simulink library "common_lib"  (R2023a)
settings: Solver=ode45  StartTime=0.0  StopTime=10.0  RelTol=1e-3
undefined symbols (not defined in the file): ACCEL_PRE_MULT, APDT_SrvcMgr_IRVHVDCSubFcnReq, C_C1GearNumbers, C_C1GearRatios, C_Calibration, C_DitherWaveform, C_GearOffset, C_GearRatioIn, C_GearRatioInverseOut, C_GearRatioOut, CLUTCH_INNER_LOOP_UPDATE_RATE, CONSTANT, DEGRADED_MODE_SIZE, Dem_EventStatusType, DiscIntNeverNeededParam, F_FAULT_ENUM, F_NOFAULT, F_OUTOFRANGE, F_RATELIMIT, FALSE, FMI14_SPECIAL_INSTRUCTIONS, FMI20_DATA_DRIFTED_HIGH, FMI21_DATA_DRIFTED_LOW, FMI29_RESERVED_FOR_SAE_ASSIGNMENT, FMI30_RESERVED_FOR_SAE_ASSIGNMENT, FMI31_CONDITION_EXISTS, FMI32_NO_FAULT, IC, k_accel, k_mean, MAX_UINT32, MEAN_PRE_MULT, NTriggers, QLTY_SIGNAL_FAILED, QLTY_SIGNAL_FULLY_FUNCTION, QLTY_SIGNAL_SUBSTITUTED_BY_1ST_CHOICE, QLTY_SIGNAL_SUBSTITUTED_BY_2ND_CHOICE, QLTY_SIGNAL_SUBSTITUTED_BY_3RD_CHOICE, QLTY_SIGNAL_SUBSTITUTED_BY_4TH_CHOICE, SAMPLE_TIME_100us, SAMPLETIME_10ms_Int, SATURATION_U16, simin, T_TestPoint, TF_FALSE, TF_TRUE, TimeStep, TRUE, WORKSPACE_UPDATE_RATE, ZERO, Zero
libraries: $bdroot x123, simulink x28, simulink_extras x4, MBD_EPS_Local_Blockset x4
(part 9 of 10)

== system common_lib/Diag/Fault Counter/FaultCounter ==
  fl : Inport
  count_prev : Inport  Port=2
  fc_level : Inport  Port=3
  reset : Inport  Port=4  OutDataTypeStr=boolean
  Enable : EnablePort  ZeroCross=off
  Constant1 : Constant  Value=ZERO
  Constant2 : Constant  Value=false
  Constant3 : Constant  Value=true
  Constant6 : Constant  Value=ZERO
  Relay : $bdroot/Slink/Relay  init=false
      settings: AttributesFormatString=ic=%<init>
  Sat : $bdroot/Slink/Sat
  Sum : Sum  Inputs=++|  InputSameDT=on  OutDataTypeStr=Inherit: Same as first input
  reset switch1 : Switch  Criteria=u2 ~= 0  Threshold=0.5  ZeroCross=off  SaturateOnIntegerOverflow=off
  count : Outport  OutputWhenDisabled=reset  InitialOutput=ZERO  VectorParamsAs1DForOutWhenUnconnected=off
  fc : Outport  Port=2  OutputWhenDisabled=reset  InitialOutput=false  VectorParamsAs1DForOutWhenUnconnected=off
  wires:
  Sum/1 -> reset switch1/3
  Constant6/1 -> reset switch1/1
  Relay/1 -> fc/1
  Constant3/1 -> Relay/4
  Constant2/1 -> Relay/5
  Constant1/1 -> Relay/3, Sat/3
  fc_level/1 -> Relay/2, Sat/2
  fl/1 -> Sum/2
  reset/1 -> reset switch1/2
  reset switch1/1 -> Relay/1, Sat/1
  count_prev/1 -> Sum/1
  Sat/1 -> count/1

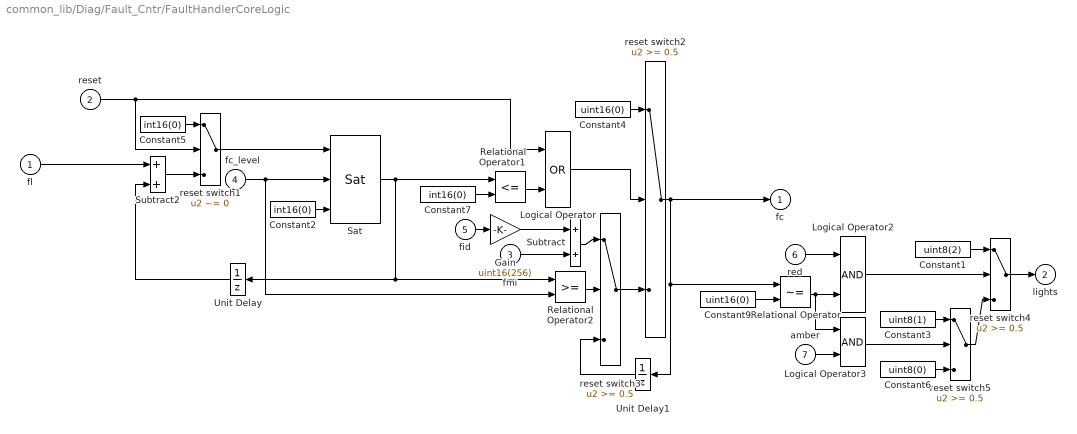
== system common_lib/Diag/Fault_Cntr/FaultHandlerCoreLogic ==
  fl : Inport  OutDataTypeStr=int16
  reset : Inport  Port=2  OutDataTypeStr=boolean
  fmi : Inport  Port=3  OutDataTypeStr=uint16
  fc_level : Inport  Port=4  OutDataTypeStr=int16
  fid : Inport  Port=5  OutDataTypeStr=uint16
  red : Inport  Port=6  OutDataTypeStr=boolean
  amber : Inport  Port=7  OutDataTypeStr=boolean
  Constant1 : Constant  Value=uint8(2)
  Constant2 : Constant  Value=int16(0)
  Constant3 : Constant  Value=uint8(1)
  Constant4 : Constant  Value=uint16(0)
  Constant5 : Constant  Value=int16(0)
  Constant6 : Constant  Value=uint8(0)
  Constant7 : Constant  Value=int16(0)
  Constant9 : Constant  Value=uint16(0)
  Gain : Gain  Gain=uint16(256)
  Logical Operator : Logic  Operator=OR  AllPortsSameDT=off  OutDataTypeStr=boolean
  Logical Operator2 : Logic  AllPortsSameDT=off  OutDataTypeStr=boolean
  Logical Operator3 : Logic  AllPortsSameDT=off  OutDataTypeStr=boolean
  Relational Operator : RelationalOperator  Operator=~=  OutDataTypeStr=boolean  InputSameDT=off
  Relational Operator1 : RelationalOperator  Operator=<=  OutDataTypeStr=boolean  InputSameDT=off
  Relational Operator2 : RelationalOperator  OutDataTypeStr=boolean  InputSameDT=off
  Sat : $bdroot/Slink/Sat
  Subtract : Sum  OutDataTypeStr=uint16
  Subtract2 : Sum  OutDataTypeStr=int16  SaturateOnIntegerOverflow=on
  Unit Delay : UnitDelay  InitialCondition=int16(0)  SampleTime=-1  HasFrameUpgradeWarning=on
      settings: AttributesFormatString=ic=%<X0>
  Unit Delay1 : UnitDelay  InitialCondition=uint16(0)  SampleTime=-1  HasFrameUpgradeWarning=on
      settings: AttributesFormatString=ic=%<X0>
  reset switch1 : Switch  Criteria=u2 ~= 0  Threshold=0.5  ZeroCross=off  SaturateOnIntegerOverflow=off
  reset switch{2..5} (4 alike) : Switch  Threshold=0.5  ZeroCross=off  SaturateOnIntegerOverflow=off
  fc : Outport  VectorParamsAs1DForOutWhenUnconnected=off
  lights : Outport  Port=2  VectorParamsAs1DForOutWhenUnconnected=off
  wires:
  Gain/1 -> Subtract/1
  reset switch3/1 -> reset switch2/3
  Unit Delay1/1 -> reset switch3/3
  Relational Operator2/1 -> reset switch3/2
  Relational Operator1/1 -> Logical Operator/2
  Constant7/1 -> Relational Operator1/2
  Unit Delay/1 -> Subtract2/2
  Subtract2/1 -> reset switch1/3
  reset switch1/1 -> Sat/1
  Constant5/1 -> reset switch1/1
  reset switch2/1 -> Unit Delay1/1, Relational Operator/1, fc/1
  Logical Operator/1 -> reset switch2/2
  Subtract/1 -> reset switch3/1
  Constant4/1 -> reset switch2/1
  fmi/1 -> Subtract/2
  fid/1 -> Gain/1
  reset/1 -> Logical Operator/1, reset switch1/2
  fl/1 -> Subtract2/1
  Sat/1 -> Relational Operator2/1, Unit Delay/1, Relational Operator1/1
  Constant9/1 -> Relational Operator/2
  Logical Operator2/1 -> reset switch4/2
  Relational Operator/1 -> Logical Operator2/2, Logical Operator3/1
  red/1 -> Logical Operator2/1
  amber/1 -> Logical Operator3/2
  fc_level/1 -> Sat/2, Relational Operator2/2
  Constant2/1 -> Sat/3
  Constant1/1 -> reset switch4/1
  Logical Operator3/1 -> reset switch5/2
  reset switch5/1 -> reset switch4/3
  Constant3/1 -> reset switch5/1
  Constant6/1 -> reset switch5/3
  reset switch4/1 -> lights/1

== system common_lib/Diag/Filter w Fault Handler/FilterWithFaultHandlerCoreLogic ==
  note: Common Library::Diagnostics::Filter With Fault Handler
  input : Inport
  tau : Inport  Port=2
  override_value : Inport  Port=3
  override? : Inport  Port=4
  reset? : Inport  Port=5
  default : Inport  Port=6
  ramp_time : Inport  Port=7
  fault? : Inport  Port=8
  Abs1 : Abs  ZeroCross=off  SaturateOnIntegerOverflow=off
  Abs2 : Abs  ZeroCross=off  SaturateOnIntegerOverflow=off
  Constant5 : Constant  Value=TimeStep
  Data Type Conversion : DataTypeConversion  OutDataTypeStr=single  SaturateOnIntegerOverflow=off  RndMeth=Floor
  Fltr_wRO : $bdroot/Fltrs/Fltr_wRO  TimeStep=TimeStep
  Product1 : Product  Inputs=**/  InputSameDT=on  OutDataTypeStr=Inherit: Same as first input
  Sum1 : Sum  Inputs=+-|  InputSameDT=on  OutDataTypeStr=Inherit: Same as first input
  Sum2 : Sum  Inputs=+-|  InputSameDT=on  OutDataTypeStr=Inherit: Same as first input
  Sum3 : Sum  Inputs=+-|  InputSameDT=on  OutDataTypeStr=Inherit: Same as first input
  Switch{1..4} (4 alike) : Switch  Threshold=0.5  ZeroCross=off  SaturateOnIntegerOverflow=off
  delay : UnitDelay  InitialCondition=Zero  SampleTime=-1  HasFrameUpgradeWarning=on
  ic: signal at fault : UnitDelay  InitialCondition=Zero  SampleTime=-1  HasFrameUpgradeWarning=on
  within zero tol of corrections : RelationalOperator  Operator=<  ZeroCross=off  InputSameDT=off
  output : Outport  VectorParamsAs1DForOutWhenUnconnected=off
  wires:
  Data Type Conversion/1 -> Product1/2
  Constant5/1 -> Data Type Conversion/1
  Sum3/1 -> Abs1/1
  delay/1 -> Switch2/1
  Switch3/1 -> delay/1
  within zero tol of corrections/1 -> Switch3/2
  Abs2/1 -> within zero tol of corrections/1
  Abs1/1 -> within zero tol of corrections/2
  Sum2/1 -> Switch3/1
  Switch1/1 -> Sum3/1, Sum2/1
  Switch4/1 -> Switch1/3, Sum1/1, ic: signal at fault/1
  ic: signal at fault/1 -> Switch4/1
  Product1/1 -> Abs2/1, Sum2/2
  Sum1/1 -> Product1/1
  default/1 -> Sum3/2, Switch3/3, Sum1/2
  Fltr_wRO/1 -> Switch4/3, output/1
  input/1 -> Switch2/3
  Switch2/1 -> Switch1/1, Fltr_wRO/1
  reset?/1 -> Fltr_wRO/5
  override?/1 -> Fltr_wRO/4
  override_value/1 -> Fltr_wRO/3
  tau/1 -> Fltr_wRO/2
  fault?/1 -> Switch1/2, Switch4/2, Switch2/2
  ramp_time/1 -> Product1/3

== system common_lib/Diag/Filter w Fault Handler1/Fltr_wRO ==
  note: This is a simple 1st order filter block with reset and override.
      |
      |      If override is true (1) then output=override_value
      |      If       reset is true (1) then output=input
      |    otherwise output = previous output + (input - previous output) * T/tau
  note: Common Library::Filters::Filter with Reset and Override
  input : Inport
  tau : Inport  Port=2
  reset? : Inport  Port=3  OutDataTypeStr=boolean
  Constant1 : Constant  Value=TimeStep
  Constant3 : Constant  Value=TimeStep
  MinMax : MinMax  Function=max  Inputs=2  InputSameDT=on  SaturateOnIntegerOverflow=on  ZeroCross=off
  Product : Product  Inputs=**/  InputSameDT=on  OutDataTypeStr=Inherit: Same as first input
  Sum : Sum  Inputs=|+-  InputSameDT=on  OutDataTypeStr=Inherit: Same as first input
  Sum1 : Sum  Inputs=|++  InputSameDT=on  OutDataTypeStr=Inherit: Same as first input
  Switch2 : Switch  Threshold=0.5  ZeroCross=off  SaturateOnIntegerOverflow=off
  Unit Delay : UnitDelay  InitialCondition=IC  SampleTime=-1  HasFrameUpgradeWarning=on
  output : Outport  VectorParamsAs1DForOutWhenUnconnected=off
  wires:
  Sum1/1 -> Switch2/3
  Product/1 -> Sum1/1
  tau/1 -> MinMax/2
  Constant1/1 -> MinMax/1
  Unit Delay/1 -> Sum1/2, Sum/2
  input/1 -> Switch2/1, Sum/1
  Constant3/1 -> Product/2
  MinMax/1 -> Product/3
  reset?/1 -> Switch2/2
  Sum/1 -> Product/1
  Switch2/1 -> Unit Delay/1, output/1

== system common_lib/Diagnostics/CAN OOR Fault Detection/detect fault ==
  In1 : Inport
  Enable : EnablePort
  Data Type Conversion Inherited : simulink/Signal Attributes/Data Type Conversion Inherited  ConvertRealWorld=Real World Value  RndMeth=Ceiling  DoSatur=off
  Data Type Conversion Inherited1 : simulink/Signal Attributes/Data Type Conversion Inherited  ConvertRealWorld=Real World Value  RndMeth=Ceiling  DoSatur=off
  Logical Operator : Logic  Operator=OR  AllPortsSameDT=off  OutDataTypeStr=boolean
  Relational Operator : RelationalOperator  Operator=<  OutDataTypeStr=boolean  ZeroCross=off  InputSameDT=off
  Relational Operator1 : RelationalOperator  Operator=<  OutDataTypeStr=boolean  ZeroCross=off  InputSameDT=off
  max : Constant  Value=k_max
  min : Constant  Value=k_min
  fault set : Outport
  wires:
  Relational Operator1/1 -> Logical Operator/1
  Relational Operator/1 -> Logical Operator/2
  Logical Operator/1 -> fault set/1
  Data Type Conversion Inherited/1 -> Relational Operator1/1
  Data Type Conversion Inherited1/1 -> Relational Operator/2
  min/1 -> Data Type Conversion Inherited1/2
  max/1 -> Data Type Conversion Inherited/2
  In1/1 -> Data Type Conversion Inherited1/1, Relational Operator1/2, Relational Operator/1, Data Type Conversion Inherited/1

== system common_lib/Diagnostics/Calibration Enabled MinMax OOR/Enabled OOR ==
  In : Inport
  ULim : Inport  Port=2
  LLim : Inport  Port=3
  Ext_Fault : Inport  Port=4
  Enable : EnablePort  ZeroCross=off
      settings: AttributesFormatString=%<StatesWhenEnabling>
  Calibration with Pretty Print Value : $bdroot/IO/Calibration with Pretty Print Value  CalValue=C_IMgmt_OOR_MinMaxCapture_Enable  scaling=None
  OOR Fault Detection : $bdroot/Diag/OOR Fault Detection  InitialValue=InitialValue
  OOR MinMax Capture : Subsystem
  Out : Outport  InitialOutput=0  VectorParamsAs1DForOutWhenUnconnected=off
      settings: AttributesFormatString=|
      | OutputWhenDisabled=%<OutputWhenDisabled>
      | InitialOutput=%<InitialOutput>
  Fault : Outport  Port=2  InitialOutput=0  VectorParamsAs1DForOutWhenUnconnected=off
      settings: AttributesFormatString=|
      | OutputWhenDisabled=%<OutputWhenDisabled>
      | InitialOutput=%<InitialOutput>
  Max : Outport  Port=3  VectorParamsAs1DForOutWhenUnconnected=off
      settings: AttributesFormatString=|
      | OutputWhenDisabled=%<OutputWhenDisabled>
      | InitialOutput=%<InitialOutput>
  Min : Outport  Port=4  VectorParamsAs1DForOutWhenUnconnected=off
      settings: AttributesFormatString=|
      | OutputWhenDisabled=%<OutputWhenDisabled>
      | InitialOutput=%<InitialOutput>
  wires:
  LLim/1 -> OOR Fault Detection/3
  ULim/1 -> OOR Fault Detection/2
  In/1 -> OOR Fault Detection/1, OOR MinMax Capture/1(Input)
  Ext_Fault/1 -> OOR Fault Detection/4, OOR MinMax Capture/2(Hold)
  OOR Fault Detection/1 -> Out/1
  OOR Fault Detection/2 -> Fault/1
  OOR MinMax Capture/1(Max) -> Max/1
  OOR MinMax Capture/2(Min) -> Min/1
  Calibration with Pretty Print Value/1 -> OOR MinMax Capture/Enable

== system common_lib/Diagnostics/Calibration Enabled MinMax RLim/Enabled RLim ==
  In : Inport
  RLim : Inport  Port=2
  Ext_Fault : Inport  Port=3
  Enable : EnablePort  ZeroCross=off
      settings: AttributesFormatString=%<StatesWhenEnabling>
  Calibration with Pretty Print Value : $bdroot/IO/Calibration with Pretty Print Value  CalValue=C_IMgmt_RLim_MinMaxCapture_Enable  scaling=None
  Data Type Conversion : DataTypeConversion  OutDataTypeStr=single  SaturateOnIntegerOverflow=off  RndMeth=Floor
  Data Type Conversion1 : DataTypeConversion  OutDataTypeStr=single  SaturateOnIntegerOverflow=off  RndMeth=Floor
  RLim MinMax Capture : Subsystem
  RateLimit : Subsystem  mask{IC=IC, TimeStep=TimeStep}
      mask prompts: IC "Initial Condition"; TimeStep "Update Time"
  out : Outport  VectorParamsAs1DForOutWhenUnconnected=off
      settings: AttributesFormatString=|
      | OutputWhenDisabled=%<OutputWhenDisabled>
      | InitialOutput=%<InitialOutput>
  fault? : Outport  Port=2  VectorParamsAs1DForOutWhenUnconnected=off
      settings: AttributesFormatString=|
      | OutputWhenDisabled=%<OutputWhenDisabled>
      | InitialOutput=%<InitialOutput>
  Max Pos Rate : Outport  Port=3  VectorParamsAs1DForOutWhenUnconnected=off
      settings: AttributesFormatString=|
      | OutputWhenDisabled=%<OutputWhenDisabled>
      | InitialOutput=%<InitialOutput>
  Max Neg Rate : Outport  Port=4  VectorParamsAs1DForOutWhenUnconnected=off
      settings: AttributesFormatString=|
      | OutputWhenDisabled=%<OutputWhenDisabled>
      | InitialOutput=%<InitialOutput>
  wires:
  In/1 -> Data Type Conversion/1, RLim MinMax Capture/1(Input)
  Ext_Fault/1 -> RLim MinMax Capture/2(Hold), RateLimit/3(ext_fault?)
  RateLimit/1(out) -> out/1
  RLim/1 -> Data Type Conversion1/1
  RateLimit/2(fault?) -> fault?/1
  RLim MinMax Capture/2(Min) -> Max Neg Rate/1
  RLim MinMax Capture/1(Max) -> Max Pos Rate/1
  Data Type Conversion/1 -> RateLimit/1(in)
  Data Type Conversion1/1 -> RateLimit/2(rlim)
  Calibration with Pretty Print Value/1 -> RLim MinMax Capture/Enable

== system common_lib/Diagnostics/DiagDbncCntr/Counter1 ==
  note: Counter increments when "incr condition" is TRUE and decrements when "decr condition" is TRUE.
  note: Common Library::Miscellaneous::Counter
  up_val : Inport
  count_up? : Inport  Port=2  OutDataTypeStr=boolean
  down_val : Inport  Port=3
  count_down? : Inport  Port=4  OutDataTypeStr=boolean
  max_count : Inport  Port=5
  min_count : Inport  Port=6
  reset? : Inport  Port=7  OutDataTypeStr=boolean
  Constant1 : Constant  Value=Zero  OutDataTypeStr=uint16
  Constant2 : Constant  Value=Zero  OutDataTypeStr=uint16
  Constant4 : Constant  Value=IC
  Constant5 : Constant  Value=false
  Logical Operator : Logic  Operator=OR
  Sat : $bdroot/Slink/Sat
  Sum : Sum  Inputs=++-  InputSameDT=on  SaturateOnIntegerOverflow=on  OutDataTypeStr=Inherit: Same as first input
  Unit Delay : UnitDelay  InitialCondition=IC  SampleTime=-1  HasFrameUpgradeWarning=on
  Unit Delay1 : UnitDelay  InitialCondition=true  SampleTime=-1  HasFrameUpgradeWarning=on
  dec switch : Switch  Threshold=0.5  ZeroCross=off  SaturateOnIntegerOverflow=off
  inc switch : Switch  Threshold=0.5  ZeroCross=off  SaturateOnIntegerOverflow=off
  reset switch : Switch  Threshold=0.5  ZeroCross=off  SaturateOnIntegerOverflow=off
  output : Outport  VectorParamsAs1DForOutWhenUnconnected=off
  wires:
  count_down?/1 -> dec switch/2
  down_val/1 -> dec switch/1
  count_up?/1 -> inc switch/2
  up_val/1 -> inc switch/1
  Constant2/1 -> dec switch/3
  dec switch/1 -> Sum/3
  Constant1/1 -> inc switch/3
  inc switch/1 -> Sum/2
  reset?/1 -> Logical Operator/1
  reset switch/1 -> Unit Delay/1, output/1
  Unit Delay/1 -> Sum/1
  Logical Operator/1 -> reset switch/2
  Unit Delay1/1 -> Logical Operator/2
  Constant5/1 -> Unit Delay1/1
  Sat/1 -> reset switch/3
  Constant4/1 -> reset switch/1
  max_count/1 -> Sat/2
  min_count/1 -> Sat/3
  Sum/1 -> Sat/1

== system common_lib/Diagnostics/OOR Fault Detect Enum/detect fault ==
  In1 : Inport
  Enable : EnablePort
  Logical Operator : Logic  Operator=OR  AllPortsSameDT=off  OutDataTypeStr=boolean
  Relational Operator : RelationalOperator  Operator=<  OutDataTypeStr=boolean  ZeroCross=off  InputSameDT=off
  Relational Operator1 : RelationalOperator  Operator=<  OutDataTypeStr=boolean  ZeroCross=off  InputSameDT=off
  max : Constant  Value=k_max
  min : Constant  Value=k_min
  fault set : Outport
  wires:
  Relational Operator1/1 -> Logical Operator/1
  Relational Operator/1 -> Logical Operator/2
  In1/1 -> Relational Operator1/2, Relational Operator/1
  Logical Operator/1 -> fault set/1
  max/1 -> Relational Operator1/1
  min/1 -> Relational Operator/2

== system common_lib/Diagnostics/OOR Fault Detection/detect fault ==
  In1 : Inport
  Enable : EnablePort
  Data Type Conversion Inherited : simulink/Signal Attributes/Data Type Conversion Inherited  ConvertRealWorld=Real World Value  DoSatur=off
  Data Type Conversion Inherited1 : simulink/Signal Attributes/Data Type Conversion Inherited  ConvertRealWorld=Real World Value  DoSatur=off
  Logical Operator : Logic  Operator=OR  AllPortsSameDT=off
  Relational Operator : RelationalOperator  Operator=<  ZeroCross=off  InputSameDT=off
  Relational Operator1 : RelationalOperator  Operator=<  ZeroCross=off  InputSameDT=off
  max : Constant  Value=k_max
  min : Constant  Value=k_min
  fault set : Outport
  wires:
  Logical Operator/1 -> fault set/1
  In1/1 -> Data Type Conversion Inherited1/1, Relational Operator/1, Relational Operator1/2, Data Type Conversion Inherited/1
  Relational Operator/1 -> Logical Operator/2
  Relational Operator1/1 -> Logical Operator/1
  max/1 -> Data Type Conversion Inherited/2
  Data Type Conversion Inherited/1 -> Relational Operator1/1
  min/1 -> Data Type Conversion Inherited1/2
  Data Type Conversion Inherited1/1 -> Relational Operator/2

== system common_lib/Diagnostics/SetFMI/IF_ELSE_LADDER ==
  FMI_in : Inport  OutDataTypeStr=uint8  PortDimensions=1
  Active1 : Inport  Port=2  OutDataTypeStr=boolean  PortDimensions=1
  Active2 : Inport  Port=3  OutDataTypeStr=boolean  PortDimensions=1
  Active3 : Inport  Port=4  OutDataTypeStr=boolean  PortDimensions=1
  Active4 : Inport  Port=5  OutDataTypeStr=boolean  PortDimensions=1
  Active5 : Inport  Port=6  OutDataTypeStr=boolean  PortDimensions=1
  Active6 : Inport  Port=7  OutDataTypeStr=boolean  PortDimensions=1
  Active7 : Inport  Port=8  OutDataTypeStr=boolean  PortDimensions=1
  FMI_1 : Inport  Port=9  OutDataTypeStr=uint8  PortDimensions=1
  FMI_2 : Inport  Port=10  OutDataTypeStr=uint8  PortDimensions=1
  FMI_3 : Inport  Port=11  OutDataTypeStr=uint8  PortDimensions=1
  FMI_4 : Inport  Port=12  OutDataTypeStr=uint8  PortDimensions=1
  FMI_5 : Inport  Port=13  OutDataTypeStr=uint8  PortDimensions=1
  FMI_6 : Inport  Port=14  OutDataTypeStr=uint8  PortDimensions=1
  FMI_7 : Inport  Port=15  OutDataTypeStr=uint8  PortDimensions=1
  Constant1 : Constant  Value=FMI32_NO_FAULT
  Constant7 : Constant  Value=FMI32_NO_FAULT
  Relational Operator : RelationalOperator  Operator=~=  OutDataTypeStr=boolean  InputSameDT=off
  Switch{,1..7} (8 alike) : Switch  Threshold=0.5  SaturateOnIntegerOverflow=off  InputSameDT=off
  FMI_out : Outport  OutDataTypeStr=uint8  PortDimensions=1  VectorParamsAs1DForOutWhenUnconnected=off
  wires:
  Constant1/1 -> Switch7/3
  FMI_in/1 -> Relational Operator/1, Switch/1
  Active6/1 -> Switch6/2
  Switch1/1 -> Switch/3
  FMI_2/1 -> Switch2/1
  Switch4/1 -> Switch3/3
  FMI_5/1 -> Switch5/1
  Switch3/1 -> Switch2/3
  Switch6/1 -> Switch5/3
  Switch/1 -> FMI_out/1
  FMI_4/1 -> Switch4/1
  FMI_7/1 -> Switch7/1
  FMI_3/1 -> Switch3/1
  Switch7/1 -> Switch6/3
  Active4/1 -> Switch4/2
  Switch5/1 -> Switch4/3
  Constant7/1 -> Relational Operator/2
  Switch2/1 -> Switch1/3
  Active2/1 -> Switch2/2
  Active7/1 -> Switch7/2
  Active1/1 -> Switch1/2
  Active3/1 -> Switch3/2
  Active5/1 -> Switch5/2
  FMI_6/1 -> Switch6/1
  FMI_1/1 -> Switch1/1
  Relational Operator/1 -> Switch/2

== system common_lib/Diagnostics/SignalSubstitution/If Action Subsystem ==
  NoSubstitute : Inport
  Action Port : ActionPort
  Constant4 : Constant  Value=QLTY_SIGNAL_FULLY_FUNCTION  SampleTime=-1
  Signal Conversion : SignalConversion  OverrideOpt=off
  Signal : Outport  VectorParamsAs1DForOutWhenUnconnected=off
  Qlty : Outport  Port=2  VectorParamsAs1DForOutWhenUnconnected=off
  wires:
  NoSubstitute/1 -> Signal Conversion/1
  Constant4/1 -> Qlty/1
  Signal Conversion/1 -> Signal/1

== system common_lib/Diagnostics/SignalSubstitution/If Action Subsystem1 ==
  FirstChoice : Inport
  Action Port : ActionPort
  Constant4 : Constant  Value=QLTY_SIGNAL_SUBSTITUTED_BY_1ST_CHOICE  SampleTime=-1
  Signal Conversion : SignalConversion  OverrideOpt=off
  Signal : Outport  VectorParamsAs1DForOutWhenUnconnected=off
  Qlty : Outport  Port=2  VectorParamsAs1DForOutWhenUnconnected=off
  wires:
  Constant4/1 -> Qlty/1
  FirstChoice/1 -> Signal Conversion/1
  Signal Conversion/1 -> Signal/1

== system common_lib/Diagnostics/SignalSubstitution/If Action Subsystem2 ==
  SecondChoice : Inport
  Action Port : ActionPort
  Constant4 : Constant  Value=QLTY_SIGNAL_SUBSTITUTED_BY_2ND_CHOICE  SampleTime=-1
  Signal Conversion : SignalConversion  OverrideOpt=off
  Signal : Outport  VectorParamsAs1DForOutWhenUnconnected=off
  Qlty : Outport  Port=2  VectorParamsAs1DForOutWhenUnconnected=off
  wires:
  Signal Conversion/1 -> Signal/1
  SecondChoice/1 -> Signal Conversion/1
  Constant4/1 -> Qlty/1

== system common_lib/Diagnostics/SignalSubstitution/If Action Subsystem3 ==
  ThirdChoice : Inport
  Action Port : ActionPort
  Constant4 : Constant  Value=QLTY_SIGNAL_SUBSTITUTED_BY_3RD_CHOICE  SampleTime=-1
  Signal Conversion : SignalConversion  OverrideOpt=off
  Signal : Outport  VectorParamsAs1DForOutWhenUnconnected=off
  Qlty : Outport  Port=2  VectorParamsAs1DForOutWhenUnconnected=off
  wires:
  Constant4/1 -> Qlty/1
  ThirdChoice/1 -> Signal Conversion/1
  Signal Conversion/1 -> Signal/1

== system common_lib/Diagnostics/SignalSubstitution/If Action Subsystem4 ==
  FourthChoice : Inport
  Action Port : ActionPort
  Constant4 : Constant  Value=QLTY_SIGNAL_SUBSTITUTED_BY_4TH_CHOICE  SampleTime=-1
  Signal Conversion : SignalConversion  OverrideOpt=off
  Signal : Outport  VectorParamsAs1DForOutWhenUnconnected=off
  Qlty : Outport  Port=2  VectorParamsAs1DForOutWhenUnconnected=off
  wires:
  Signal Conversion/1 -> Signal/1
  FourthChoice/1 -> Signal Conversion/1
  Constant4/1 -> Qlty/1

== system common_lib/Diagnostics/SignalSubstitution/If Action Subsystem5 ==
  FailedValue : Inport
  Action Port : ActionPort
  Constant4 : Constant  Value=QLTY_SIGNAL_FAILED  SampleTime=-1
  Signal Conversion : SignalConversion  OverrideOpt=off
  Signal : Outport  VectorParamsAs1DForOutWhenUnconnected=off
  Qlty : Outport  Port=2  VectorParamsAs1DForOutWhenUnconnected=off
  wires:
  Constant4/1 -> Qlty/1
  FailedValue/1 -> Signal Conversion/1
  Signal Conversion/1 -> Signal/1

== system common_lib/Fltrs/Fltr_wRO/FilterCoreLogic ==
  note: This is a simple 1st order filter block
  input : Inport  OutDataTypeStr=single
  tau : Inport  Port=2  OutDataTypeStr=single
  override_value : Inport  Port=3
  override? : Inport  Port=4  OutDataTypeStr=boolean
  reset? : Inport  Port=5  OutDataTypeStr=boolean
  Constant1 : Constant  Value=Ts
  MinMax : MinMax  Function=max  Inputs=2  InputSameDT=on  SaturateOnIntegerOverflow=on  ZeroCross=off
  Product : Product  Inputs=**/  InputSameDT=on  OutDataTypeStr=Inherit: Same as first input
  Sum : Sum  Inputs=|+-  InputSameDT=on  OutDataTypeStr=Inherit: Same as first input
  Sum1 : Sum  Inputs=|++  InputSameDT=on  OutDataTypeStr=Inherit: Same as first input
  Switch : Switch  Threshold=0.5  ZeroCross=off  SaturateOnIntegerOverflow=off
  Switch2 : Switch  Threshold=0.5  ZeroCross=off  SaturateOnIntegerOverflow=off
  Unit Delay : UnitDelay  InitialCondition=IC  SampleTime=-1  HasFrameUpgradeWarning=on
  output : Outport  OutDataTypeStr=single  VectorParamsAs1DForOutWhenUnconnected=off
  wires:
  Sum1/1 -> Switch2/3
  Product/1 -> Sum1/1
  tau/1 -> MinMax/2
  input/1 -> Sum/1, Switch2/1
  MinMax/1 -> Product/3
  Sum/1 -> Product/1
  Constant1/1 -> MinMax/1, Product/2
  override_value/1 -> Switch/1
  override?/1 -> Switch/2
  Switch/1 -> output/1, Unit Delay/1
  reset?/1 -> Switch2/2
  Switch2/1 -> Switch/3
  Unit Delay/1 -> Sum1/2, Sum/2

== system common_lib/Fltrs/Fltr_wROExtInitCond/FilterCoreLogic ==
  note: This is a simple 1st order filter block
  input : Inport  OutDataTypeStr=single
  tau : Inport  Port=2  OutDataTypeStr=single
  init_cond : Inport  Port=3  OutDataTypeStr=single
  task_rate : Inport  Port=4  OutDataTypeStr=single
  reset : Inport  Port=5  OutDataTypeStr=boolean
  override : Inport  Port=6  OutDataTypeStr=boolean
  override_value : Inport  Port=7
  ClampAboveZero : $bdroot/Misc/ClampAboveZero  Tol=single(1e-9)
      settings: AttributesFormatString=tol=%<Tol>
  Constant : Constant  Value=FALSE  SampleTime=-1
  MinMax : MinMax  Function=max  Inputs=2  InputSameDT=on  SaturateOnIntegerOverflow=on  ZeroCross=off
  Product : Product  Inputs=**/  InputSameDT=on  SaturateOnIntegerOverflow=on  OutDataTypeStr=Inherit: Same as first input
  Sum : Sum  Inputs=|+-  InputSameDT=on  SaturateOnIntegerOverflow=on  OutDataTypeStr=Inherit: Same as first input
  Sum1 : Sum  Inputs=|++  InputSameDT=on  SaturateOnIntegerOverflow=on  OutDataTypeStr=Inherit: Same as first input
  Switch : Switch  Threshold=0.5  ZeroCross=off
  Switch1 : Switch  Criteria=u2 ~= 0  Threshold=0.5  ZeroCross=off
  Switch2 : Switch  Threshold=0.5  ZeroCross=off
  Unit Delay : UnitDelay  InitialCondition=TRUE  SampleTime=-1  HasFrameUpgradeWarning=on
      settings: AttributesFormatString=ic=%<X0>
  Unit Delay1 : UnitDelay  InitialCondition=single(0)  SampleTime=-1  HasFrameUpgradeWarning=on
      settings: AttributesFormatString=ic=%<X0>
  output : Outport  OutDataTypeStr=single  VectorParamsAs1DForOutWhenUnconnected=off
  wires:
  Switch1/1 -> Sum1/2, Sum/2
  Sum1/1 -> Switch2/3
  Product/1 -> Sum1/1
  tau/1 -> MinMax/2
  input/1 -> Switch2/1, Sum/1
  MinMax/1 -> ClampAboveZero/1
  Sum/1 -> Product/1
  task_rate/1 -> Product/2, MinMax/1
  override_value/1 -> Switch/1
  override/1 -> Switch/2
  Switch/1 -> output/1
  reset/1 -> Switch2/2
  Switch2/1 -> Unit Delay1/1, Switch/3
  Constant/1 -> Unit Delay/1
  Unit Delay/1 -> Switch1/2
  init_cond/1 -> Switch1/1
  Unit Delay1/1 -> Switch1/3
  ClampAboveZero/1 -> Product/3

== system common_lib/Fltrs/Int16FIR/Accum ==
  Buf : Inport
  Constant : Constant  Value=int16(2*N-2)
  Constant1 : Constant  Value=int16(N-1)
  Data Type Conversion : DataTypeConversion  OutDataTypeStr=int32  SaturateOnIntegerOverflow=off  RndMeth=Floor
  Data Type Conversion1 : DataTypeConversion  OutDataTypeStr=int32  SaturateOnIntegerOverflow=off  RndMeth=Floor
  Demux : Demux  Outputs=2
  For Iterator : ForIterator  ResetStates=reset  IterationLimit=N-1  IndexMode=Zero-based  IterationVariableDataType=int16
  Mux : Mux  Inputs=2
  Product : Product  OutDataTypeStr=int32
  Selector : Selector  IndexMode=Zero-based  InputPortWidth=2*N  IndexOptions=Index vector (port)  Indices=[1 3]  OutputSizes=1
  Sum : Sum  Inputs=++|  AccumDataTypeStr=int32  OutDataTypeStr=int32
  Sum1 : Sum  Inputs=|+-
  Sum2 : Sum  Inputs=|+-
  Sum3 : Sum  Inputs=|+-
  Sum4 : Sum  Inputs=+++  AccumDataTypeStr=int32  OutDataTypeStr=int32
  Unit Delay : UnitDelay  SampleTime=-1  HasFrameUpgradeWarning=on
  Unit Delay1 : UnitDelay  SampleTime=-1  HasFrameUpgradeWarning=on
  Accel_Accum : Outport  VectorParamsAs1DForOutWhenUnconnected=off
  Mean_Accum : Outport  Port=2  VectorParamsAs1DForOutWhenUnconnected=off
  wires:
  Unit Delay1/1 -> Sum4/1
  Demux/1 -> Sum1/1, Sum4/2
  Sum4/1 -> Unit Delay1/1, Mean_Accum/1
  Data Type Conversion1/1 -> Product/1
  Data Type Conversion/1 -> Demux/1
  Sum3/1 -> Mux/2
  Product/1 -> Sum/2
  Sum2/1 -> Data Type Conversion1/1
  Constant1/1 -> Sum2/1
  Sum1/1 -> Product/2
  Demux/2 -> Sum4/3, Sum1/2
  Unit Delay/1 -> Sum/1
  Selector/1 -> Data Type Conversion/1
  Buf/1 -> Selector/1
  Mux/1 -> Selector/2
  Constant/1 -> Sum3/1
  For Iterator/1 -> Sum3/2, Mux/1, Sum2/2
  Sum/1 -> Unit Delay/1, Accel_Accum/1

== system common_lib/Gear Ratios/FindGearNumberByRatio/Timer1 ==
  In : Inport
  TriggerTime : Inport  Port=2
  Data Type Conversion : DataTypeConversion  OutDataTypeStr=single  SaturateOnIntegerOverflow=off  RndMeth=Floor
  Discrete-Time Integrator : DiscreteIntegrator  gainval=single(1.0)  ExternalReset=falling  InitialCondition=single(0)  SampleTime=TimeStep  LimitOutput=on  ICPrevOutput=DiscIntNeverNeededParam  ICPrevScaledInput=DiscIntNeverNeededParam
  Relational Operator : RelationalOperator  Operator=>  OutDataTypeStr=boolean  InputSameDT=off
  Signal Specification : SignalSpecification  OutDataTypeStr=boolean
  Out : Outport  VectorParamsAs1DForOutWhenUnconnected=off
  wires:
  Relational Operator/1 -> Out/1
  TriggerTime/1 -> Relational Operator/2
  Discrete-Time Integrator/1 -> Relational Operator/1
  Data Type Conversion/1 -> Discrete-Time Integrator/1
  In/1 -> Signal Specification/1
  Signal Specification/1 -> Data Type Conversion/1, Discrete-Time Integrator/2

== system common_lib/Misc/EdgeTriggered Pulse w time/EdgeTriggeredPulseCoreLogic ==
  note: Initial Condition
  note: Common Library::Miscellaneous::Edge Triggered Pulse with Time
  input : Inport  OutDataTypeStr=boolean
  width : Inport  Port=2  OutDataTypeStr=single
  And : Logic
  Constant2 : Constant  Value=true
  Constant3 : Constant  Value=false
  Logical Operator1 : Logic  Operator=OR
  Not : Logic  Operator=NOT
  Relational Operator1 : RelationalOperator  Operator=>  ZeroCross=off
  Sample Rate : Constant  Value=Ts
  Sample Rate Half : Constant  Value=Ts_half
  Sum : Sum  Inputs=|++  InputSameDT=on  SaturateOnIntegerOverflow=on  OutDataTypeStr=Inherit: Same as first input
  Sum1 : Sum  Inputs=-+|  InputSameDT=on  SaturateOnIntegerOverflow=on  OutDataTypeStr=Inherit: Same as first input
  Switch : Switch  Threshold=0.5  ZeroCross=off
  Switch1 : Switch  Threshold=0.5  ZeroCross=off
  Switch2 : Switch  Threshold=0.5  ZeroCross=off
  Unit Delay1 : UnitDelay  InitialCondition=true  SampleTime=-1  HasFrameUpgradeWarning=on
      settings: AttributesFormatString=ic=%<X0>
  Unit Delay2 : UnitDelay  InitialCondition=single(0)  SampleTime=-1  HasFrameUpgradeWarning=on
      settings: AttributesFormatString=ic=%<X0>
  Unit Delay4 : UnitDelay  InitialCondition=true  SampleTime=-1  HasFrameUpgradeWarning=on
      settings: AttributesFormatString=ic=%<X0>
  pulse : Outport  OutDataTypeStr=boolean  VectorParamsAs1DForOutWhenUnconnected=off
  wires:
  input/1 -> And/1, Unit Delay1/1
  Sample Rate/1 -> Switch/1, Sum/1
  Constant3/1 -> Switch2/1
  Unit Delay4/1 -> Logical Operator1/2, Switch2/3
  Switch2/1 -> Switch1/3
  Constant2/1 -> Switch1/1
  Switch1/1 -> Unit Delay4/1, pulse/1
  Relational Operator1/1 -> Switch1/2
  And/1 -> Switch2/2, Logical Operator1/1
  Logical Operator1/1 -> Switch/2
  Unit Delay2/1 -> Sum/2
  Sum/1 -> Switch/3
  Sum1/1 -> Relational Operator1/1
  Not/1 -> And/2
  Unit Delay1/1 -> Not/1
  Switch/1 -> Unit Delay2/1, Sum1/2
  width/1 -> Relational Operator1/2
  Sample Rate Half/1 -> Sum1/1

== system common_lib/Misc/Timeout Detection/TimeoutLogic ==
  Change : Inport
  Timeout : Inport  Port=2
  MinMax : MinMax  Inputs=2  InputSameDT=on  SaturateOnIntegerOverflow=on  ZeroCross=off
  Sample Rate : Constant  Value=Ts
  Sample Rate Tolerance : Constant  Value=Tol
  Sum : Sum  Inputs=++|  InputSameDT=on  OutDataTypeStr=Inherit: Same as first input
  Sum1 : Sum  Inputs=-+|  InputSameDT=on  OutDataTypeStr=Inherit: Same as first input
  Switch : Switch  Threshold=0.5  ZeroCross=off  SaturateOnIntegerOverflow=off
  Unit Delay : UnitDelay  InitialCondition=Zero  SampleTime=-1  HasFrameUpgradeWarning=on
  zero : Constant  Value=Zero
  time : Outport  VectorParamsAs1DForOutWhenUnconnected=off
  wires:
  Unit Delay/1 -> Sum/1
  MinMax/1 -> Unit Delay/1
  zero/1 -> Switch/3
  Switch/1 -> Sum1/2, MinMax/2
  Sum/1 -> Switch/1
  Timeout/1 -> MinMax/1
  Sample Rate/1 -> Sum/2
  Sample Rate Tolerance/1 -> Sum1/1
  Sum1/1 -> time/1
  Change/1 -> Switch/2

== system common_lib/Misc/Timeout with time/TimeoutLogic ==
  Change : Inport
  Timeout : Inport  Port=2
  MinMax : MinMax  Inputs=2  InputSameDT=on  SaturateOnIntegerOverflow=on  ZeroCross=off
  Sample Rate : Constant  Value=Ts
  Sample Rate Tolerance : Constant  Value=Tol
  Sum : Sum  Inputs=++|  InputSameDT=on  SaturateOnIntegerOverflow=on  OutDataTypeStr=Inherit: Same as first input
  Sum1 : Sum  Inputs=-+|  InputSameDT=on  SaturateOnIntegerOverflow=on  OutDataTypeStr=Inherit: Same as first input
  Switch : Switch  Threshold=0.5  ZeroCross=off
  Unit Delay : UnitDelay  InitialCondition=Zero  SampleTime=-1  HasFrameUpgradeWarning=on
      settings: AttributesFormatString=%<InitialCondition>
  zero : Constant  Value=Zero
  time : Outport  VectorParamsAs1DForOutWhenUnconnected=off
  wires:
  Change/1 -> Switch/2
  Sum1/1 -> time/1
  Sample Rate Tolerance/1 -> Sum1/1
  Sample Rate/1 -> Sum/2
  Timeout/1 -> MinMax/1
  Sum/1 -> Switch/1
  Switch/1 -> MinMax/2, Sum1/2
  zero/1 -> Switch/3
  MinMax/1 -> Unit Delay/1
  Unit Delay/1 -> Sum/1

== system common_lib/Misc/Timeout with time Integer/TimeoutLogic ==
  Change : Inport
  Timeout : Inport  Port=2
  Data Type Conversion : DataTypeConversion  OutDataTypeStr=uint16  RndMeth=Floor
  MinMax : MinMax  Inputs=2  InputSameDT=on  SaturateOnIntegerOverflow=on  ZeroCross=off
  Sample Rate : Constant  Value=Ts
  Sample Rate Tolerance : Constant  Value=Tol
  Sum : Sum  Inputs=++|  InputSameDT=on  SaturateOnIntegerOverflow=on  OutDataTypeStr=Inherit: Same as first input
  Sum1 : Sum  Inputs=-+|  InputSameDT=on  SaturateOnIntegerOverflow=on  OutDataTypeStr=Inherit: Same as first input
  Switch : Switch  Threshold=0.5  ZeroCross=off
  Unit Delay : UnitDelay  InitialCondition=Zero  SampleTime=-1  HasFrameUpgradeWarning=on
      settings: AttributesFormatString=%<InitialCondition>
  zero : Constant  Value=Zero
  time : Outport  VectorParamsAs1DForOutWhenUnconnected=off
  wires:
  Unit Delay/1 -> Sum/1
  MinMax/1 -> Unit Delay/1
  zero/1 -> Switch/3
  Switch/1 -> Sum1/2, MinMax/2
  Sum/1 -> Switch/1
  Timeout/1 -> MinMax/1
  Sample Rate/1 -> Data Type Conversion/1
  Sample Rate Tolerance/1 -> Sum1/1
  Sum1/1 -> time/1
  Change/1 -> Switch/2
  Data Type Conversion/1 -> Sum/2

== system common_lib/OS/Scheduler with Init/Init Relay ==
  Task 1 : TriggerPort  TriggerType=function-call  VariantControl=(inherit)  StatesWhenEnabling=reset  ZeroCross=off
  Constant2 : Constant  Value=FALSE
  Function Call : Subsystem  TreatAsAtomicUnit=on
  Unit Delay2 : UnitDelay  InitialCondition=TRUE  SampleTime=-1  HasFrameUpgradeWarning=on
      settings: AttributesFormatString=ic=%<X0>
  Init : Outport  VectorParamsAs1DForOutWhenUnconnected=off
  wires:
  Function Call/1(Init) -> Init/1
  Constant2/1 -> Unit Delay2/1
  Unit Delay2/1 -> Function Call/Enable

== system common_lib/Signal Conditioning/HydValveDither/CalculateActualFreq ==
  desired_freqency_hz : Inport
  sample_time : Inport  Port=2
  ClampAroundZero : $bdroot/Misc/ClampAroundZero  Tol=single(eps)
      settings: AttributesFormatString=tol=%<Tol>
  ClampAroundZero1 : $bdroot/Misc/ClampAroundZero  Tol=single(eps)
      settings: AttributesFormatString=tol=%<Tol>
  Constant4 : Constant  Value=single(0)
  Constant7 : Constant  Value=single(1)
  Constant8 : Constant  Value=single(1)
  Product4 : Product  RndMeth=Zero
  Product5 : Product  Inputs=*/  RndMeth=Zero
  Product6 : Product  RndMeth=Zero
  Product7 : Product  Inputs=*/  RndMeth=Zero
  Rounding Function : Rounding  Operator=round
  Switch : Switch  Criteria=u2 > Threshold  SaturateOnIntegerOverflow=off  InputSameDT=off
  realized_freq : Outport  VectorParamsAs1DForOutWhenUnconnected=off
  sample_times_per_cycle : Outport  Port=2  VectorParamsAs1DForOutWhenUnconnected=off
  wires:
  sample_time/1 -> Product4/1, Product6/1
  Constant7/1 -> Product5/1
  Product5/1 -> Rounding Function/1, sample_times_per_cycle/1  "sample_times_per_period"
  Rounding Function/1 -> Product6/2
  Constant8/1 -> Product7/1
  Product6/1 -> ClampAroundZero1/1
  desired_freqency_hz/1 -> Product4/2, Switch/2
  Product4/1 -> ClampAroundZero/1
  ClampAroundZero/1 -> Product5/2
  ClampAroundZero1/1 -> Product7/2
  Product7/1 -> Switch/1
  Switch/1 -> realized_freq/1
  Constant4/1 -> Switch/3

== system common_lib/Signal Conditioning/HydValveDither/TableBasedSignalGen ==
  sample_times_per_cycle : Inport
  Constant1 : Constant  Value=single(32768)
  Constant5 : Constant  Value=int32(1)
  Constant6 : Constant  Value=length(DitherWaveform)-1  OutDataTypeStr=uint16
  Constant9 : Constant  Value=length(DitherWaveform)-1  OutDataTypeStr=single
  Data Type Conversion2 : DataTypeConversion  OutDataTypeStr=uint16  RndMeth=Nearest  SaturateOnIntegerOverflow=off
  Data Type Conversion3 : DataTypeConversion  OutDataTypeStr=int32  RndMeth=Nearest  SaturateOnIntegerOverflow=off
  Direct Lookup Table (n-D) : LookupNDDirect  NumberOfTableDimensions=1  Table=DitherWaveform
  Discrete-Time Integrator : DiscreteIntegrator  IntegratorMethod=Accumulation: Forward Euler  ExternalReset=rising  SampleTime=ts  ShowStatePort=on  ICPrevOutput=DiscIntNeverNeededParam  ICPrevScaledInput=DiscIntNeverNeededParam
  MinMax : MinMax  Inputs=2
  MinMax1 : MinMax  Inputs=2
  Product8 : Product  Inputs=*/*  RndMeth=Zero
  Relational Operator : RelationalOperator  Operator=<=  OutDataTypeStr=boolean  InputSameDT=off
  out : Outport  VectorParamsAs1DForOutWhenUnconnected=off
  wires:
  Discrete-Time Integrator/1 -> Product8/1
  Relational Operator/1 -> [reset_integrator]
  [reset_integrator] -> Discrete-Time Integrator/2
  Product8/1 -> Data Type Conversion2/1
  Discrete-Time Integrator/State -> Relational Operator/2
  Constant5/1 -> Discrete-Time Integrator/1
  Data Type Conversion3/1 -> Relational Operator/1
  Constant9/1 -> Product8/3
  Constant6/1 -> MinMax/2
  Data Type Conversion2/1 -> MinMax/1
  MinMax/1 -> Direct Lookup Table (n-D)/1
  Direct Lookup Table (n-D)/1 -> out/1
  sample_times_per_cycle/1 -> Product8/2, MinMax1/2
  MinMax1/1 -> Data Type Conversion3/1
  Constant1/1 -> MinMax1/1

== system common_lib/Signal Conditioning/Obsolete Signal Conditioning/BooleanToTernary ==
  note: Boolean to Ternary Conversion
      | Eaton Corporation
  Boolean : Inport
  Constant1 : Constant  Value=TF_TRUE
  Constant4 : Constant  Value=TF_FALSE
  Switch : Switch  Threshold=0.5  ZeroCross=off  SaturateOnIntegerOverflow=off  InputSameDT=off
  Ternary : Outport  VectorParamsAs1DForOutWhenUnconnected=off
  wires:
  Boolean/1 -> Switch/2
  Switch/1 -> Ternary/1
  Constant4/1 -> Switch/3
  Constant1/1 -> Switch/1

== system common_lib/Signal Conditioning/Obsolete Signal Conditioning/Ternary To Boolean (Default False) ==
  note: Ternary To Boolean Conversion (Default False)
      | Eaton Corporation
  note: Outputs a FALSE upon an invalid or FALSE input
      | Outputs a TRUE upon a TRUE (149) input
  Ternary : Inport
  Constant1 : Constant  Value=TF_TRUE
  Data Type Conversion : DataTypeConversion  OutDataTypeStr=uint8  SaturateOnIntegerOverflow=off
  Relational Operator : RelationalOperator  Operator===  ZeroCross=off  InputSameDT=off
  Boolean : Outport  VectorParamsAs1DForOutWhenUnconnected=off
  wires:
  Ternary/1 -> Data Type Conversion/1
  Relational Operator/1 -> Boolean/1
  Constant1/1 -> Relational Operator/1
  Data Type Conversion/1 -> Relational Operator/2

== system common_lib/Signal Conditioning/Obsolete Signal Conditioning/Ternary To Boolean (Default True) ==
  note: Outputs a TRUE upon an invalid or TRUE input
      | Outputs a FALSE upon a FALSE (89) input
  note: Ternary To Boolean Conversion (Default True)
      | Eaton Corporation
  Ternary : Inport
  Constant1 : Constant  Value=TF_FALSE
  Data Type Conversion : DataTypeConversion  OutDataTypeStr=uint8  SaturateOnIntegerOverflow=off
  Relational Operator : RelationalOperator  Operator=~=  ZeroCross=off  InputSameDT=off
  Boolean : Outport  VectorParamsAs1DForOutWhenUnconnected=off
  wires:
  Data Type Conversion/1 -> Relational Operator/2
  Constant1/1 -> Relational Operator/1
  Relational Operator/1 -> Boolean/1
  Ternary/1 -> Data Type Conversion/1

== system common_lib/Signal Generators/Clu_2_1_3_1_1_1_TestSignalBuilder/TestFrequencyRamp ==
  TestFreqRampStartFreq : Inport
  TestFreqRampEndFreq : Inport  Port=2
  TestFreqRampTime : Inport  Port=3
  TestSignalEnable : Inport  Port=4
  Test_Reset : Inport  Port=5
  ClampAroundZero2 : $bdroot/Misc/ClampAroundZero  Tol=single(eps(1))
      settings: AttributesFormatString=tol=%<Tol>
  Constant1 : Constant  Value=CLUTCH_INNER_LOOP_UPDATE_RATE
  Constant3 : Constant  Value=ZERO
  Constant30 : Constant  Value=ZERO
  Constant4 : Constant  Value=ZERO
  Data Type Conversion : DataTypeConversion  OutDataTypeStr=single  SaturateOnIntegerOverflow=off
  Integrator2 : $bdroot/Ctrl/Integrator  TimeStep=CLUTCH_INNER_LOOP_UPDATE_RATE  IC=single(0.0)
  Product6 : Product  Inputs=*/*  InputSameDT=on  OutDataTypeStr=Inherit: Same as first input
  Sum3 : Sum  Inputs=+-|  InputSameDT=on  OutDataTypeStr=Inherit: Same as first input
  Sum5 : Sum  Inputs=|++  InputSameDT=on  OutDataTypeStr=Inherit: Same as first input
  Switch1 : Switch  Threshold=0.5  ZeroCross=off  SaturateOnIntegerOverflow=off  InputSameDT=off
  TestFreqRampFreq : Outport  InitialOutput=[single(0)]  VectorParamsAs1DForOutWhenUnconnected=off
      settings: AttributesFormatString=InitialOutput=%<InitialOutput>\nOutputWhenDisabled=%<OutputWhenDisabled>
  wires:
  TestFreqRampEndFreq/1 -> Sum3/1, [TgtFreq]
  TestFreqRampStartFreq/1 -> Sum3/2, [InitFreq]
  Sum3/1 -> Product6/1
  TestFreqRampTime/1 -> ClampAroundZero2/1
  Constant30/1 -> Integrator2/4
  [TgtFreq] -> Integrator2/2
  Constant4/1 -> Integrator2/3
  Integrator2/1 -> Sum5/1
  Sum5/1 -> TestFreqRampFreq/1  "TestFreqRampFreq"
  [InitFreq] -> Sum5/2
  Switch1/1 -> Integrator2/1
  Product6/1 -> Switch1/1
  Constant3/1 -> Switch1/3
  ClampAroundZero2/1 -> Product6/2
  TestSignalEnable/1 -> Switch1/2
  Test_Reset/1 -> Integrator2/5
  Constant1/1 -> Data Type Conversion/1
  Data Type Conversion/1 -> Product6/3

== system common_lib/Signal Generators/Clu_2_1_3_1_1_1_TestSignalBuilder/TestOffsetRamp ==
  TestWaveOffsetRampStart : Inport
  TestWaveOffsetRampEnd : Inport  Port=2
  TestWaveOffsetRampTime : Inport  Port=3
  Test_Enable : Inport  Port=4
  Test_Reset : Inport  Port=5
  ClampAroundZero1 : $bdroot/Misc/ClampAroundZero  Tol=single(eps(1))
      settings: AttributesFormatString=tol=%<Tol>
  Constant11 : Constant  Value=ZERO
  Constant8 : Constant  Value=ZERO
  Constant9 : Constant  Value=ZERO
  Integrator3 : $bdroot/Ctrl/Integrator  TimeStep=CLUTCH_INNER_LOOP_UPDATE_RATE  IC=single(0.0)
  Product4 : Product  Inputs=*/  InputSameDT=on  OutDataTypeStr=Inherit: Same as first input
  Sum7 : Sum  Inputs=+-|  InputSameDT=on  OutDataTypeStr=Inherit: Same as first input
  Switch3 : Switch  Threshold=0.5  ZeroCross=off  SaturateOnIntegerOverflow=off  InputSameDT=off
  TestConstant : Outport  InitialOutput=[single(0)]  VectorParamsAs1DForOutWhenUnconnected=off
      settings: AttributesFormatString=InitialOutput=%<InitialOutput>\nOutputWhenDisabled=%<OutputWhenDisabled>
  TestOffsetRamp : Outport  Port=2  InitialOutput=[single(0)]  VectorParamsAs1DForOutWhenUnconnected=off
      settings: AttributesFormatString=InitialOutput=%<InitialOutput>\nOutputWhenDisabled=%<OutputWhenDisabled>
  wires:
  TestWaveOffsetRampStart/1 -> Sum7/2
  Sum7/1 -> Product4/1
  TestWaveOffsetRampTime/1 -> ClampAroundZero1/1
  Constant9/1 -> Integrator3/4
  [TestWaveOffsetRampEnd] -> Integrator3/2
  Constant11/1 -> Integrator3/3
  Switch3/1 -> Integrator3/1
  Product4/1 -> Switch3/1
  Constant8/1 -> Switch3/3
  ClampAroundZero1/1 -> Product4/2
  Integrator3/1 -> TestOffsetRamp/1
  TestWaveOffsetRampEnd/1 -> Sum7/1, [TestWaveOffsetRampEnd], TestConstant/1
  Test_Enable/1 -> Switch3/2
  Test_Reset/1 -> Integrator3/5

== system common_lib/Signal Generators/Clu_2_1_3_1_1_1_TestSignalBuilder/TestRampWaves ==
  TestOffsetRamp : Inport
  TestWave : Inport  Port=2
  TestWaveSignSwitch : Inport  Port=3
  Constant : Constant  Value=single(0.0)  SampleTime=-1
  EdgeTriggered Pulse : $bdroot/Misc/EdgeTriggered Pulse  Edge=FALSE to TRUE  Width=single(CLUTCH_INNER_LOOP_UPDATE_RATE)  Pulse=TRUE  TimeStep=CLUTCH_INNER_LOOP_UPDATE_RATE  Init=0
  Hold : $bdroot/Misc/Hold  SystemSampleTime=-1  VariantActivationTime=update diagram  Latency=0  AutoFrameSizeCalculation=off
  Relational Operator : RelationalOperator  Operator=>  ZeroCross=off  InputSameDT=off
  Sum1 : Sum  InputSameDT=on  OutDataTypeStr=Inherit: Same as first input
  Sum2 : Sum  InputSameDT=on  OutDataTypeStr=Inherit: Same as first input
  SineWave : Outport  VectorParamsAs1DForOutWhenUnconnected=off
  SquareWave : Outport  Port=2  VectorParamsAs1DForOutWhenUnconnected=off
  wires:
  Sum1/1 -> SineWave/1
  TestOffsetRamp/1 -> Hold/1, Sum1/1
  TestWave/1 -> Sum1/2, Sum2/2
  TestWaveSignSwitch/1 -> Relational Operator/1
  EdgeTriggered Pulse/1 -> Hold/Enable
  Hold/1 -> Sum2/1
  Sum2/1 -> SquareWave/1
  Relational Operator/1 -> EdgeTriggered Pulse/1
  Constant/1 -> Relational Operator/2

== system common_lib/Signal Generators/Clu_2_1_3_1_1_1_TestSignalBuilder/TestWaveCreation ==
  note: Outputtype
      | 0. Constant
      | 1. Ramp
      | 2. Sine Wave
      | 3. Square Wave
      | 4. Zero
  TestFreqRampFreq : Inport
  TestWaveAmplitude : Inport  Port=2
  Test_Reset : Inport  Port=3
  CluPresCmdTestSignalType : Inport  Port=4
  Constant1 : Constant  Value=-1
  Constant10 : Constant  Value=pi/2.0
  Constant12 : Constant  Value=-1.0
  Constant13 : Constant  Value=1.0
  Constant2 : Constant  Value=single(0.0)
  Constant3 : Constant  Value=single(0.0)
  Constant30 : Constant  Value=ZERO
  Constant4 : Constant  Value=single(0.0)
  Data Type Conversion{12..13,19..20} (4 alike) : DataTypeConversion  OutDataTypeStr=single  SaturateOnIntegerOverflow=off
  Integrator1 : $bdroot/Ctrl/Integrator  TimeStep=CLUTCH_INNER_LOOP_UPDATE_RATE  IC=single(0.0)
  Multiport Switch : MultiPortSwitch  DataPortOrder=Zero-based contiguous  Inputs=4  DataPortForDefault=Additional data port  zeroidx=on  SaturateOnIntegerOverflow=off  InputSameDT=off
  Product1 : Product  Inputs=**  InputSameDT=on  OutDataTypeStr=Inherit: Same as first input
  Product2 : Product  Inputs=**  InputSameDT=on  OutDataTypeStr=Inherit: Same as first input
  Product5 : Product  Inputs=**  InputSameDT=on  OutDataTypeStr=Inherit: Same as first input
  Relay : $bdroot/Slink/Relay  init=single(1.0)
  Sine1 : $bdroot/Misc/Sine
  Unit Delay4 : UnitDelay  InitialCondition=single(1.0)  SampleTime=-1  HasFrameUpgradeWarning=on
      settings: AttributesFormatString=ic=%<X0>
  TestWave : Outport  InitialOutput=[single(0)]  VectorParamsAs1DForOutWhenUnconnected=off
      settings: AttributesFormatString=InitialOutput=%<InitialOutput>\nOutputWhenDisabled=%<OutputWhenDisabled>
  TestWaveSignSwitch : Outport  Port=2  InitialOutput=[single(0)]  VectorParamsAs1DForOutWhenUnconnected=off
      settings: AttributesFormatString=InitialOutput=%<InitialOutput>\nOutputWhenDisabled=%<OutputWhenDisabled>
  wires:
  Constant12/1 -> Data Type Conversion19/1
  Constant13/1 -> Data Type Conversion20/1
  Data Type Conversion19/1 -> Relay/4
  Data Type Conversion20/1 -> Relay/5
  Relay/1 -> Unit Delay4/1, Multiport Switch/5, TestWaveSignSwitch/1
  Unit Delay4/1 -> [TestWaveSignSwitch]
  Integrator1/1 -> Relay/1, Sine1/1
  TestWaveAmplitude/1 -> Product2/1
  Product2/1 -> TestWave/1
  [TestWaveSignSwitch] -> Product5/2
  Product5/1 -> Integrator1/1  "ChirpFrequency"
  Constant10/1 -> Data Type Conversion12/1, Product1/1
  Product1/1 -> Data Type Conversion13/1
  Constant1/1 -> Product1/2
  Data Type Conversion12/1 -> Integrator1/2, Relay/2
  Data Type Conversion13/1 -> Integrator1/3, Relay/3
  Constant30/1 -> Integrator1/4
  Test_Reset/1 -> Integrator1/5
  TestFreqRampFreq/1 -> Product5/1
  CluPresCmdTestSignalType/1 -> Multiport Switch/1
  Constant2/1 -> Multiport Switch/2
  Constant3/1 -> Multiport Switch/3
  Constant4/1 -> Multiport Switch/6
  Multiport Switch/1 -> Product2/2
  Sine1/1 -> Multiport Switch/4
